simulink model "planning"  (R2020b)
settings: Solver=FixedStepDiscrete  StartTime=0.0  StopTime=10.0  FixedStep=0.1  RelTol=1e-3  EnableMultiTasking=on
settings Model: Creator=ana  LastModifiedBy=ana
settings SolverCC: AutoInsertRateTranBlk=on
settings DataIOCC: LimitDataPoints=on
settings OptimizationCC: LifeSpan=inf
settings DebuggingCC: AllowSymbolicDim=off  SFUnexpectedBacktrackingDiag=warning  SFNoUnconditionalDefaultTransitionDiag=warning  SFExecutionAtInitializationDiag=none  ArithmeticOperatorsInVariantConditions=warning
settings SFSimCC: SimUseLocalCustomCode=off  CustomCodeUndefinedFunction=UseInterfaceOnly
settings RTWCC: RTWUseLocalCustomCode=off
settings CodeAppCC: StateflowObjectComments=on
settings GRTTargetCC: TargetLangStandard=C89/C90 (ANSI)
settings ConfigComp: CovMetricSettings=dw  CovSaveCumulativeToWorkspaceVar=on  CovSaveSingleToWorkspaceVar=on  CovExternalEMLEnable=off

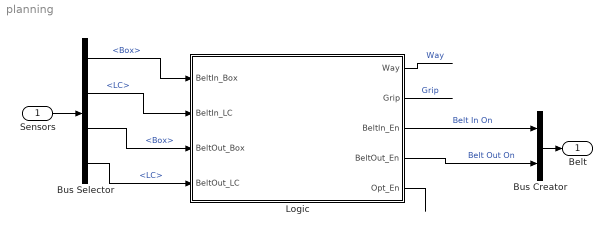
== system planning ==
  Sensors : Inport
  Bus Creator : BusCreator  Inputs=2
  Bus Selector : BusSelector  OutputSignals=Belts.BeltIn.Box,Belts.BeltIn.LC,Belts.BeltOut.Box,Belts.BeltOut.LC
  Logic : Stateflow chart  Tag=PublishSubsystem  TreatAsAtomicUnit=on  mask(Supervisory Logic for Arm, Gripper, and Belts){delayMoveBox=0.5, delayGripBox=3, delayDropBox=3.5, delayClose=3, delayBeltClear=1, delayShipBox=1.5}
      mask prompts: delayMoveBox "Delay Move Box (sec)"; delayGripBox "Delay Grip Box (sec)"; delayDropBox "Delay Drop Box (sec)"; delayClose "Delay Close Gripper at Home (sec)"; delayBeltClear "Delay Belt Clear (sec)"; delayShipBox "Delay Ship Box (sec)"
      mask help: Logic controlling robot arm, gripper, and belts. Arm movement, gripper state, and belt state are controlled based on events in the system. The parameters below are for delays that ensure actions are not triggered too early.
  Belt : Outport  VectorParamsAs1DForOutWhenUnconnected=off
  wires:
  Logic/3(BeltIn_En) -> Bus Creator/1  "Belt In On"
  Bus Creator/1 -> Belt/1
  Bus Selector/2 -> Logic/2(BeltIn_LC)  "<LC>"
  Bus Selector/4 -> Logic/4(BeltOut_LC)  "<LC>"
  Bus Selector/1 -> Logic/1(BeltIn_Box)  "<Box>"
  Bus Selector/3 -> Logic/3(BeltOut_Box)  "<Box>"
  Logic/1(Way) -> ?  "Way"
  Sensors/1 -> Bus Selector/1
  Logic/2(Grip) -> ?  "Grip"
  Logic/4(BeltOut_En) -> Bus Creator/2  "Belt Out On"
  Logic/5(Opt_En) -> ?

== stateflow chart planning/Logic ==
  state BeltIn [parallel]
    settings: executionOrder=1
    state Empty
      entry: BeltIn_En = 0;
    state On
      entry: BeltIn_En = 1;
    state BoxReady
      entry: Robot.GetBox
      BeltIn_En=0;
    state WaitClear
    (default) -> BeltIn.Empty
    (junction 133) -> BeltIn.Empty
    (junction 130) -> (junction 133)
    BeltIn.Empty -> BeltIn.On : [BeltIn_Box ==1]
    BeltIn.On -> BeltIn.BoxReady : [BeltIn_LC == 0]
    BeltIn.BoxReady -> BeltIn.WaitClear : [BeltIn_LC == 1]
    BeltIn.WaitClear -> (junction 130) : after(delayBeltClear,sec)
  state Robot [parallel]
    settings: executionOrder=2
    state StartHome
      entry: Way = 0;
    state GoBeltIn
      entry: Gripper.OpenGrip
      Way = 1;
    state BeltIn
      entry: Gripper.GripBox
    state GoBeltOut
      entry: Optimizer.CallOpt
      Way = 2;
    state BeltOut
      entry: Gripper.DropBox
    state GoingHome
      entry: Way = 3;
    state Home
      entry: Gripper.Close
    (default) -> StartHome
    StartHome -> GoBeltIn : GetBox
    (junction 138) -> GoBeltIn
    (junction 137) -> (junction 138)
    GoBeltIn -> Robot.BeltIn : after(delayGripBox,sec)
    Robot.BeltIn -> GoBeltOut : MoveBox
    GoBeltOut -> Robot.BeltOut : after(delayDropBox,sec)
    Robot.BeltOut -> GoingHome : GoHome
    GoingHome -> Home : after(delayClose,sec)
    Home -> (junction 137) : GetBox
  state Gripper [parallel]
    settings: executionOrder=3
    state Closed
      entry: Grip = 0;
    state Open
      entry: Grip = 1;
    state Tighten
      entry: Grip = 2;
    state Grip
      entry: Robot.MoveBox
    state Release
      entry: Grip = 1;
      Optimizer.OffOpt
    (default) -> Closed
    Closed -> Open : OpenGrip
    Open -> Closed [order 2] : Close
    (junction 143) -> Open
    (junction 141) -> (junction 143)
    Open -> Tighten [order 1] : GripBox
    Tighten -> Grip : after(delayMoveBox,sec)
    Grip -> Release : DropBox
    Release -> (junction 141) : [after(delayShipBox,sec)]
        | {BeltOut.ShipBox}
  state BeltOut [parallel]
    settings: executionOrder=4
    state Empty
      entry: BeltOut_En = 0;
    state WaitRelease
    state On
      entry: BeltOut_En = 1;
    state BoxReady
      entry: Robot.GoHome
      BeltOut_En = 0;
    state WaitClear
    (default) -> BeltOut.Empty
    (junction 147) -> BeltOut.Empty
    (junction 146) -> (junction 147)
    BeltOut.Empty -> WaitRelease : [BeltOut_Box == 1]
    WaitRelease -> BeltOut.On : ShipBox
    BeltOut.On -> BeltOut.BoxReady : [BeltOut_LC ==0]
    BeltOut.BoxReady -> BeltOut.WaitClear : [BeltOut_LC == 1]
    BeltOut.WaitClear -> (junction 146) : after(delayBeltClear,sec)
  state Optimizer [parallel]
    settings: executionOrder=5
    state Off
      entry: Opt_En = 0;
    state On
      entry: Opt_En = 1;
    (default) -> Off
    Off -> Optimizer.On : CallOpt
    Optimizer.On -> Off : OffOpt
  data: Way output; Grip output; BeltIn_Box input; BeltIn_LC input; BeltIn_En output; BeltOut_En output; BeltOut_Box input; BeltOut_LC input; delayClose parameter; delayDropBox parameter; delayBeltClear parameter; delayGripBox parameter; delayShipBox parameter; delayMoveBox parameter; Opt_En output
  events: GetBox local FUNCTION_CALL_EVENT; MoveBox local FUNCTION_CALL_EVENT; GoHome local FUNCTION_CALL_EVENT; OpenGrip local FUNCTION_CALL_EVENT; GripBox local FUNCTION_CALL_EVENT; DropBox local FUNCTION_CALL_EVENT; Close local FUNCTION_CALL_EVENT; ShipBox local FUNCTION_CALL_EVENT; CallOpt local FUNCTION_CALL_EVENT; OffOpt local FUNCTION_CALL_EVENT
